simulink library "model_controller"  (R2016b)
settings: Solver=VariableStepAuto  StartTime=0.0  StopTime=10.0  RelTol=1e-3
undefined symbols (not defined in the file or in its folder): acc, ad, dd, jd, jerk, snap, vel
libraries: model_controller x6, motion x1
settings Model: Creator=Dai Luyao  LastModifiedBy=Dai Luyao

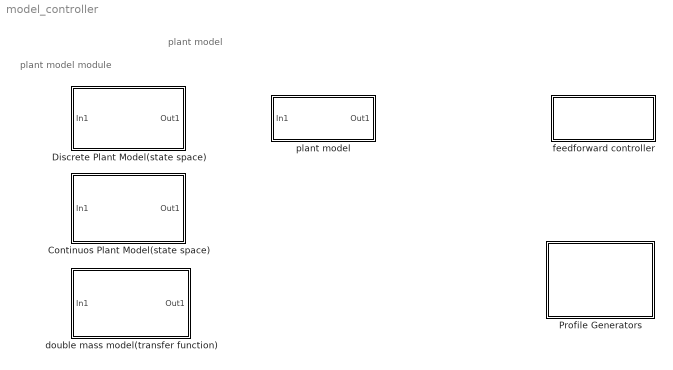
== system model_controller ==
  note: plant model
  note: plant model module
  "Continuos Plant Model(state space) " : Subsystem  mask{A=0, B=0, C=0, D=0}
  Discrete Plant Model(state space) : Subsystem  mask{A_d=0, B_d=0, C_d=0, D_d=0}
      mask prompts: A_d "A"; B_d "B"; C_d "C"; D_d "D"
  Profile Generators : Subsystem
      mask Display: disp('Profile\nGenerators')
  double mass model(transfer function) : Subsystem  mask{m1=0, m2=0, f=0, n=0}
      mask prompts: m1 "mover"; m2 "stage"; f "resonant frequency(Hz)"; n "damping ratio"
  feedforward controller : Subsystem
      mask Display: disp('feedforward controller');
  plant model : Subsystem  BlockChoice=Continuos Plant Model(state space)
      settings: TemplateBlock=self  MemberBlocks=Continuos Plant Model(state space) ,Discrete Plant Model(state space),double mass model(transfer function)

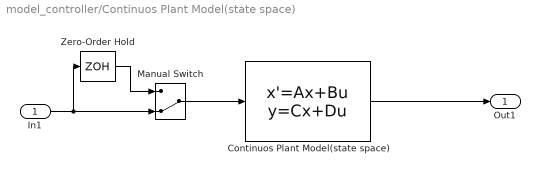
== system model_controller/Continuos Plant Model(state space)  ==
  In1 : Inport
  "Continuos Plant Model(state space) " : StateSpace  A=A  B=B  C=C  D=D  X0=0
  Manual Switch : ManualSwitch  CurrentSetting=0
  Zero-Order Hold : ZeroOrderHold  SampleTime=2e-6
  Out1 : Outport
  wires:
  "Continuos Plant Model(state space) "/1 -> Out1/1
  In1/1 -> Zero-Order Hold/1, Manual Switch/2
  Zero-Order Hold/1 -> Manual Switch/1
  Manual Switch/1 -> "Continuos Plant Model(state space) "/1

== system model_controller/Discrete Plant Model(state space) ==
  In1 : Inport
  Discrete Plant Model(state space) : DiscreteStateSpace  A=A_d  B=B_d  C=B_d  D=D_d  SampleTime=-1
  Out1 : Outport
  wires:
  In1/1 -> Discrete Plant Model(state space)/1
  Discrete Plant Model(state space)/1 -> Out1/1

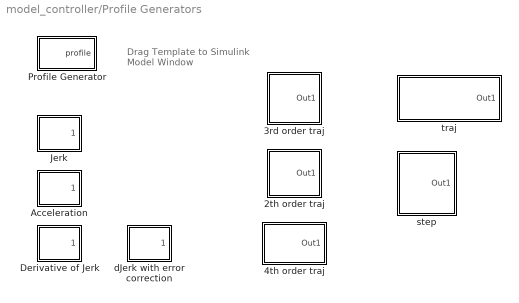
== system model_controller/Profile Generators ==
  note: Drag Template to
      | Simulink Model Window
  2th order traj : Subsystem  mask(2nd Order Profile Generator){t0=0, x=0.06, v=0.25, a=10, Ts=0}
      mask prompts: t0 "Starting time:  t0 [s]"; x "Displacement:  x [m]"; v "Bound on velocity:  vmax [m/s]"; a "Bound on acceleration:  amax [m/s2]"; Ts "Sampling time (0 for continuous):  Ts [s]"
      mask help: 2nd Order Profile Generator
      mask Help: See make2.m and look under mask
  3rd order traj : Subsystem  mask(3d Order Profile Generator){t0=0, x=0.06, v=0.25, a=10, j=800, Ts=0}
      mask prompts: t0 "Starting time:  t0 [s]"; x "Displacement:  x [m]"; v "Bound on velocity:  vmax [m/s]"; a "Bound on acceleration:  amax [m/s2]"; j "Bound on jerk: jmax [m/s3]"; Ts "Sampling time (0 for continuous):  Ts [s]"
      mask help: 3d Order Profile Generator
      mask Help: See make3.m and profile3.m and look under mask
  4th order traj : Subsystem  mask(4th Order Profile Generator){t0=0, x=0.06, v=0.25, a=10, j=800, d=64000, Ts=0}
      mask prompts: t0 "Starting time:  t0 [s]"; x "Displacement:  x [m]"; v "Bound on velocity:  vmax [m/s]"; a "Bound on acceleration:  amax [m/s2]"; j "Bound on jerk: jmax [m/s3]"; d "Bound on derivative of jerk:  dmax [m/s4]"; Ts "Sampling time (0 for continuous):  Ts [s]"
      mask help: 4th Order Profile Generator
      mask Help: See make4.m and profile4.m and look under mask
  Acceleration : Subsystem  mask(2nd Order Profile Generator){t0=.3, x=1, v=1, a=5, Ts=0}
      mask prompts: t0 "Starting time:  t0 [s]"; x "Displacement:  x [m]"; v "Bound on velocity:  vmax [m/s]"; a "Bound on acceleration:  amax [m/s2]"; Ts "Sampling time (0 for continuous):  Ts [s]"
      mask help: 2nd Order Profile Generator
      mask init:
      | [t,ad,aa,tx,a,v,p,tt] = make2(abs(x),v,a,Ts,0);
      | t0=t0-10*eps;
      mask Help: See make2.m and look under mask
      mask Display:
      | plot([0 aa(1,:)+t0],[0 aa(2,:)])
      | text(0.8*(max(aa(1,:))+t0),0,'a\n')
  Derivative of Jerk : Subsystem  mask(4th Order Profile Generator){t0=0.02, x=0.046, v=0.6, a=10, j=800, d=64000, Ts=0}
      mask prompts: t0 "Starting time:  t0 [s]"; x "Displacement:  x [m]"; v "Bound on velocity:  vmax [m/s]"; a "Bound on acceleration:  amax [m/s2]"; j "Bound on jerk: jmax [m/s3]"; d "Bound on derivative of jerk:  dmax [m/s4]"; Ts "Sampling time (0 for continuous):  Ts [s]"
      mask help: 4th Order Profile Generator
      mask init:
      | [t,dd]=make4(abs(x),v,a,j,d,Ts);
      | t0=t0-10*eps;
      | [dj,tx,d,j,a,v,p,tt]=profile4(t,dd(1),0,0);
      mask Help: See make4.m and profile4.m and look under mask
      mask Display:
      | plot([0 dj(1,:)+t0],[0 dj(2,:)])
      | text(0.8*(max(dj(1,:))+t0),0,'d\n')
  Jerk : Subsystem  mask(3d Order Profile Generator){t0=.3, x=1, v=1, a=5, j=50, Ts=0}
      mask prompts: t0 "Starting time:  t0 [s]"; x "Displacement:  x [m]"; v "Bound on velocity:  vmax [m/s]"; a "Bound on acceleration:  amax [m/s2]"; j "Bound on jerk: jmax [m/s3]"; Ts "Sampling time (0 for continuous):  Ts [s]"
      mask help: 3d Order Profile Generator
      mask init:
      | [t,jd]=make3(abs(x),v,a,j,Ts);
      | t0=t0-10*eps;
      | [jj,tx,j,a,v,p,tt]=profile3(t,jd(1),0,0);
      | global constantAccStartTime;
      | global constantAccEndTime;
      | global constantJerkStartTime;
      | global constantJerkEndTime;
      | constantAccStartTime=t0+t(1);
      | constantAccEndTime=constantAccStartTime+t(2);
      | constantJerkStartTime=t0;
      | constantJerkEndTime=t0+0.9*(t(1)-t0);
      mask Help: See make3.m and profile3.m and look under mask
      mask Display:
      | plot([0 jj(1,:)+t0],[0 jj(2,:)])
      | text(0.85*(max(jj(1,:))+t0),0,'j\n')
  Profile Generator : Subsystem  BlockChoice=Acceleration
      settings: TemplateBlock=self  MemberBlocks=Acceleration,Derivative of Jerk,Jerk,dJerk with error correction
  dJerk with error correction : Subsystem  mask(4th Order Profile Generator with quantization error correction){t0=.3, x=1, v=1, a=5, j=50, d=1000, Ts=0, r=10*eps, s=15}
      mask prompts: t0 "Starting time:  t0 [s]"; x "Displacement:  x [m]"; v "Bound on velocity:  vmax [m/s]"; a "Bound on acceleration:  amax [m/s2]"; j "Bound on jerk: jmax [m/s3]"; d "Bound on derivative of jerk:  dmax [m/s4]"; Ts "Sampling time (0 for continuous):  Ts [s]"; r "Resolution of position [m] (default: 10*eps)"; s "Number of decimals for digitized d (default: 15)"
      mask help: 4th Order Profile Generator with quantization error correction
      mask init:
      | if length(r)==0 | length(s)==0
      | 	r=10*eps;
      | 	s=15;
      | end
      | [t,dd]=make4(abs(x),v,a,j,d,Ts,r,s);
      | t0=t0-10*eps;
      | [dj,tx,d,j,a,v,p,tt]=profile4(t,dd(1),0,0);
      mask Help: See make4.m and profile4.m and look under mask
      mask Display:
      | plot([0 dj(1,:)+t0],[0 dj(2,:)])
      | text(0.8*(max(dj(1,:))+t0),0,'d\n')
  step : Subsystem  mask{t=0, v0=0, vf=1, Ts=0}
      mask prompts: t "step time:"; v0 "inital value:"; vf "final value:"; Ts "sample time"
  traj : Subsystem  BlockChoice=2th order traj
      settings: TemplateBlock=self  MemberBlocks=2th order traj,3rd order traj,4th order traj,step

== system model_controller/double mass model(transfer function) ==
  In1 : Inport
  Zero-Order Hold : ZeroOrderHold  SampleTime=-1
  double mass model(transfer function) : Subsystem
  Out1 : Outport
  wires:
  In1/1 -> Zero-Order Hold/1
  double mass model(transfer function)/1(Out1) -> Out1/1
  Zero-Order Hold/1 -> double mass model(transfer function)/1(In1)

== system model_controller/feedforward controller ==
  S-Function : S-Function  FunctionName=adaptiveFeedforward  Parameters=paraNum  SFunctionDeploymentMode=off  EnableBusSupport=off
  acceleration feedforward : Subsystem  mask{snap=snap, jerk=jerk, acc=acc, vel=vel}
      mask prompts: snap "the coefficient of snap feedforward"; jerk "the coefficient of jerk feedforward"; acc "the coefficient of acc feedforward"; vel "the coefficient of vel feedforward"
      mask Display: disp('acceleration feedforward')
  feedforward 4th order : Subsystem  mask{snap=snap, jerk=jerk, acc=acc, vel=vel}
      mask prompts: snap "the coefficient of snap feedforward"; jerk "the coefficient of jerk feedforward"; acc "the coefficient of acc feedforward"; vel "the coefficient of vel feedforward"
      mask Display: disp('acceleration feedforward')
  feedforward controller : Subsystem  BlockChoice=acceleration feedforward
      settings: TemplateBlock=self  MemberBlocks=acceleration feedforward,feedforward 4th order

== system model_controller/plant model ==
  In1 : Inport
  "Continuos Plant Model(state space) " : model_controller/Continuos Plant Model(state space)   A=0  B=0  C=0  D=0
  Out1 : Outport
  wires:
  In1/1 -> "Continuos Plant Model(state space) "/1
  "Continuos Plant Model(state space) "/1 -> Out1/1

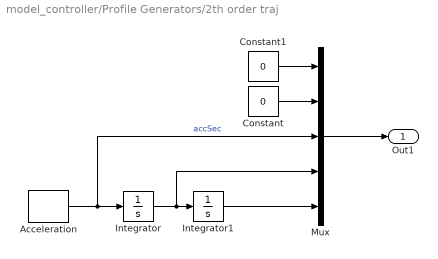
== system model_controller/Profile Generators/2th order traj ==
  Acceleration : model_controller/Profile Generators/Acceleration  t0=t0  x=x  v=v  a=a  Ts=Ts
  Constant : Constant  Value=0
  Constant1 : Constant  Value=0
  Integrator : Integrator
  Integrator1 : Integrator
  Mux : Mux  Inputs=5
  Out1 : Outport
  wires:
  Constant1/1 -> Mux/1
  Constant/1 -> Mux/2
  Integrator1/1 -> Mux/5
  Integrator/1 -> Integrator1/1, Mux/4
  Acceleration/1 -> Integrator/1, Mux/3  "accSec"
  Mux/1 -> Out1/1

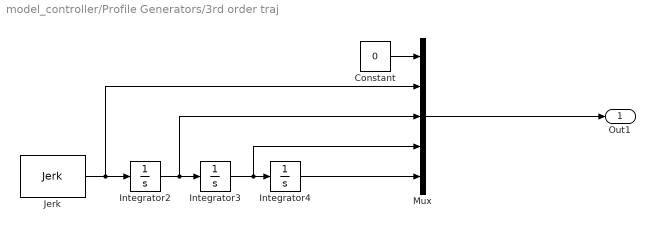
== system model_controller/Profile Generators/3rd order traj ==
  Constant : Constant  Value=0
  Integrator2 : Integrator
  Integrator3 : Integrator
  Integrator4 : Integrator
  Jerk : model_controller/Profile Generators/Jerk  t0=t0  x=x  v=v  a=a  j=j  Ts=Ts
  Mux : Mux  Inputs=5
  Out1 : Outport
  wires:
  Mux/1 -> Out1/1
  Integrator2/1 -> Mux/3, Integrator3/1
  Integrator3/1 -> Mux/4, Integrator4/1
  Jerk/1 -> Mux/2, Integrator2/1
  Integrator4/1 -> Mux/5
  Constant/1 -> Mux/1

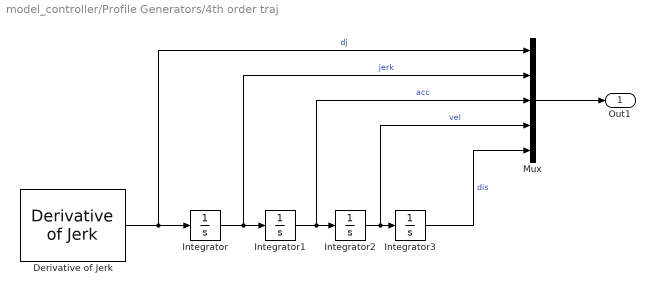
== system model_controller/Profile Generators/4th order traj ==
  Derivative of Jerk : model_controller/Profile Generators/Derivative of Jerk  t0=t0  x=x  v=v  a=a  j=j  d=d  Ts=Ts
  Integrator{,1..3} (4 alike) : Integrator
  Mux : Mux  Inputs=5
  Out1 : Outport
  wires:
  Mux/1 -> Out1/1
  Integrator/1 -> Integrator1/1, Mux/2  "jerk"
  Derivative of Jerk/1 -> Integrator/1, Mux/1  "dj"
  Integrator2/1 -> Integrator3/1, Mux/4  "vel"
  Integrator1/1 -> Integrator2/1, Mux/3  "acc"
  Integrator3/1 -> Mux/5  "dis"

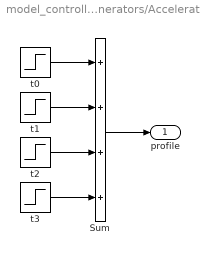
== system model_controller/Profile Generators/Acceleration ==
  Sum : Sum  Inputs=4  SaturateOnIntegerOverflow=on  InputSameDT=on  OutDataTypeStr=Inherit: Same as first input
  t0 : Step  Time=t0  After=ad(1)  SampleTime=0
  t1 : Step  Time=t0+t(1)  After=-ad(1)  SampleTime=0
  t2 : Step  Time=t0+t(1)+t(2)  After=-ad(1)  SampleTime=0
  t3 : Step  Time=t0+2*t(1)+t(2)  After=ad(1)  SampleTime=0
  profile : Outport
  wires:
  t0/1 -> Sum/1
  t1/1 -> Sum/2
  t2/1 -> Sum/3
  t3/1 -> Sum/4
  Sum/1 -> profile/1

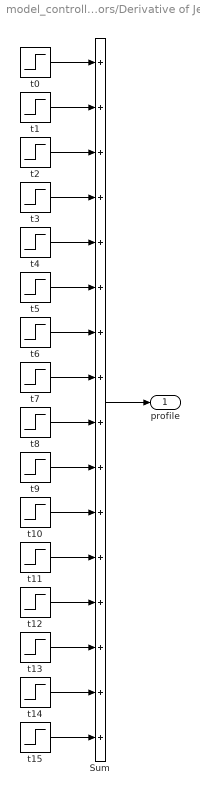
== system model_controller/Profile Generators/Derivative of Jerk ==
  Sum : Sum  Inputs=16  SaturateOnIntegerOverflow=on  InputSameDT=on  OutDataTypeStr=Inherit: Same as first input
  t0 : Step  Time=t0  After=dd(1)  SampleTime=0
  t1 : Step  Time=t0+t(1)  After=-dd(1)  SampleTime=0
  t10 : Step  Time=t0+5*t(1)+3*t(2)+t(3)+t(4)  After=dd(1)  SampleTime=0
  t11 : Step  Time=t0+6*t(1)+3*t(2)+t(3)+t(4)  After=-dd(1)  SampleTime=0
  t12 : Step  Time=t0+6*t(1)+3*t(2)+2*t(3)+t(4)  After=dd(1)  SampleTime=0
  t13 : Step  Time=t0+7*t(1)+3*t(2)+2*t(3)+t(4)  After=-dd(1)  SampleTime=0
  t14 : Step  Time=t0+7*t(1)+4*t(2)+2*t(3)+t(4)  After=-dd(1)  SampleTime=0
  t15 : Step  Time=t0+8*t(1)+4*t(2)+2*t(3)+t(4)  After=dd(1)  SampleTime=0
  t2 : Step  Time=t0+t(1)+t(2)  After=-dd(1)  SampleTime=0
  t3 : Step  Time=t0+2*t(1)+t(2)  After=dd(1)  SampleTime=0
  t4 : Step  Time=t0+2*t(1)+t(2)+t(3)  After=-dd(1)  SampleTime=0
  t5 : Step  Time=t0+3*t(1)+t(2)+t(3)  After=dd(1)  SampleTime=0
  t6 : Step  Time=t0+3*t(1)+2*t(2)+t(3)  After=dd(1)  SampleTime=0
  t7 : Step  Time=t0+4*t(1)+2*t(2)+t(3)  After=-dd(1)  SampleTime=0
  t8 : Step  Time=t0+4*t(1)+2*t(2)+t(3)+t(4)  After=-dd(1)  SampleTime=0
  t9 : Step  Time=t0+5*t(1)+2*t(2)+t(3)+t(4)  After=dd(1)  SampleTime=0
  profile : Outport
  wires:
  t0/1 -> Sum/1
  t1/1 -> Sum/2
  t2/1 -> Sum/3
  t3/1 -> Sum/4
  t4/1 -> Sum/5
  t5/1 -> Sum/6
  t6/1 -> Sum/7
  t7/1 -> Sum/8
  t8/1 -> Sum/9
  t9/1 -> Sum/10
  t10/1 -> Sum/11
  t11/1 -> Sum/12
  t12/1 -> Sum/13
  t13/1 -> Sum/14
  t14/1 -> Sum/15
  t15/1 -> Sum/16
  Sum/1 -> profile/1

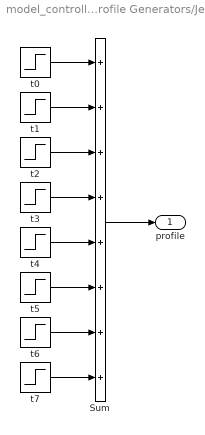
== system model_controller/Profile Generators/Jerk ==
  Sum : Sum  Inputs=8  SaturateOnIntegerOverflow=on  InputSameDT=on  OutDataTypeStr=Inherit: Same as first input
  t0 : Step  Time=t0  After=jd(1)  SampleTime=0
  t1 : Step  Time=t0+t(1)  After=-jd(1)  SampleTime=0
  t2 : Step  Time=t0+t(1)+t(2)  After=-jd(1)  SampleTime=0
  t3 : Step  Time=t0+2*t(1)+t(2)  After=jd(1)  SampleTime=0
  t4 : Step  Time=t0+2*t(1)+t(2)+t(3)  After=-jd(1)  SampleTime=0
  t5 : Step  Time=t0+3*t(1)+t(2)+t(3)  After=jd(1)  SampleTime=0
  t6 : Step  Time=t0+3*t(1)+2*t(2)+t(3)  After=jd(1)  SampleTime=0
  t7 : Step  Time=t0+4*t(1)+2*t(2)+t(3)  After=-jd(1)  SampleTime=0
  profile : Outport
  wires:
  Sum/1 -> profile/1
  t7/1 -> Sum/8
  t6/1 -> Sum/7
  t5/1 -> Sum/6
  t4/1 -> Sum/5
  t3/1 -> Sum/4
  t2/1 -> Sum/3
  t1/1 -> Sum/2
  t0/1 -> Sum/1

== system model_controller/Profile Generators/Profile Generator ==
  Acceleration : motion/Profile Generators/Acceleration  t0=.3  x=1  v=1  a=5  Ts=0
  profile : Outport
  wires:
  Acceleration/1 -> profile/1

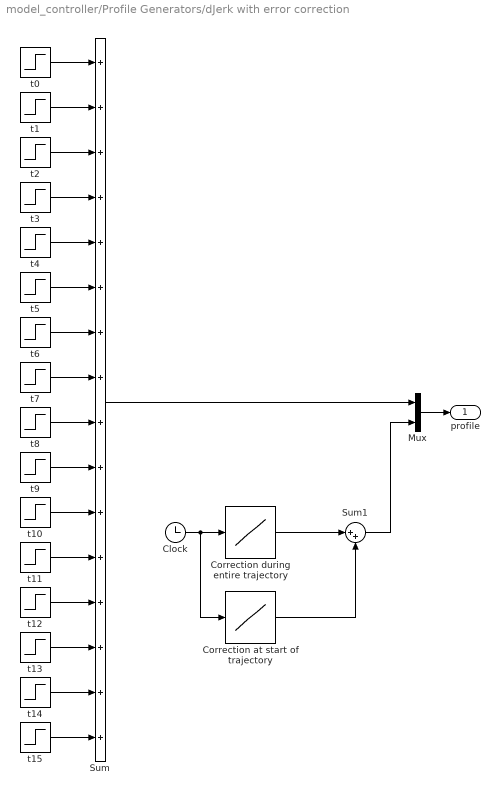
== system model_controller/Profile Generators/dJerk with error correction ==
  Clock : Clock
  Correction at start of trajectory : Lookup  InputValues="[ -1 t0 t0+abs(dd(3))*Ts  2*(t0+8*t(1)+4*t(2)+2*t(3)+t(4)) ]"  Table=[ 0 0 [1 1]*dd(3)*r]  SaturateOnIntegerOverflow=on
  Correction during entire trajectory : Lookup  InputValues="[ -1 t0  t0+8*t(1)+4*t(2)+2*t(3)+t(4)  2*(t0+8*t(1)+4*t(2)+2*t(3)+t(4)) ]"  Table=[0 0 [1 1]*dd(2)*r]  SaturateOnIntegerOverflow=on
  Mux : Mux  Inputs=2
  Sum : Sum  Inputs=16  SaturateOnIntegerOverflow=on  InputSameDT=on  OutDataTypeStr=Inherit: Same as first input
  Sum1 : Sum  Inputs=|++  SaturateOnIntegerOverflow=on  InputSameDT=on  OutDataTypeStr=Inherit: Same as first input
  t0 : Step  Time=t0  After=dd(1)  SampleTime=0
  t1 : Step  Time=t0+t(1)  After=-dd(1)  SampleTime=0
  t10 : Step  Time=t0+5*t(1)+3*t(2)+t(3)+t(4)  After=dd(1)  SampleTime=0
  t11 : Step  Time=t0+6*t(1)+3*t(2)+t(3)+t(4)  After=-dd(1)  SampleTime=0
  t12 : Step  Time=t0+6*t(1)+3*t(2)+2*t(3)+t(4)  After=dd(1)  SampleTime=0
  t13 : Step  Time=t0+7*t(1)+3*t(2)+2*t(3)+t(4)  After=-dd(1)  SampleTime=0
  t14 : Step  Time=t0+7*t(1)+4*t(2)+2*t(3)+t(4)  After=-dd(1)  SampleTime=0
  t15 : Step  Time=t0+8*t(1)+4*t(2)+2*t(3)+t(4)  After=dd(1)  SampleTime=0
  t2 : Step  Time=t0+t(1)+t(2)  After=-dd(1)  SampleTime=0
  t3 : Step  Time=t0+2*t(1)+t(2)  After=dd(1)  SampleTime=0
  t4 : Step  Time=t0+2*t(1)+t(2)+t(3)  After=-dd(1)  SampleTime=0
  t5 : Step  Time=t0+3*t(1)+t(2)+t(3)  After=dd(1)  SampleTime=0
  t6 : Step  Time=t0+3*t(1)+2*t(2)+t(3)  After=dd(1)  SampleTime=0
  t7 : Step  Time=t0+4*t(1)+2*t(2)+t(3)  After=-dd(1)  SampleTime=0
  t8 : Step  Time=t0+4*t(1)+2*t(2)+t(3)+t(4)  After=-dd(1)  SampleTime=0
  t9 : Step  Time=t0+5*t(1)+2*t(2)+t(3)+t(4)  After=dd(1)  SampleTime=0
  profile : Outport
  wires:
  Sum/1 -> Mux/1
  Mux/1 -> profile/1
  t0/1 -> Sum/1
  t1/1 -> Sum/2
  t2/1 -> Sum/3
  t3/1 -> Sum/4
  t4/1 -> Sum/5
  t5/1 -> Sum/6
  t6/1 -> Sum/7
  t7/1 -> Sum/8
  t8/1 -> Sum/9
  t9/1 -> Sum/10
  t10/1 -> Sum/11
  t11/1 -> Sum/12
  t12/1 -> Sum/13
  t13/1 -> Sum/14
  t14/1 -> Sum/15
  t15/1 -> Sum/16
  Clock/1 -> Correction during entire trajectory/1, Correction at start of trajectory/1
  Correction at start of trajectory/1 -> Sum1/2
  Sum1/1 -> Mux/2
  Correction during entire trajectory/1 -> Sum1/1

== system model_controller/Profile Generators/step ==
  Constant : Constant  Value=0
  Mux : Mux  Inputs=5
  Step : Step  Time=t  Before=v0  After=vf  SampleTime=Ts
  Out1 : Outport
  wires:
  Constant/1 -> Mux/1, Mux/4, Mux/3, Mux/2
  Mux/1 -> Out1/1
  Step/1 -> Mux/5

== system model_controller/Profile Generators/traj ==
  2th order traj : model_controller/Profile Generators/2th order traj  t0=0  x=0.06  v=0.25  a=10  Ts=0
  Out1 : Outport
  wires:
  2th order traj/1 -> Out1/1

== system model_controller/double mass model(transfer function)/double mass model(transfer function) ==
  In1 : Inport
  Transfer Fcn : TransferFcn  Denominator=[1 1]
  Out1 : Outport
  wires:
  In1/1 -> Transfer Fcn/1
  Transfer Fcn/1 -> Out1/1

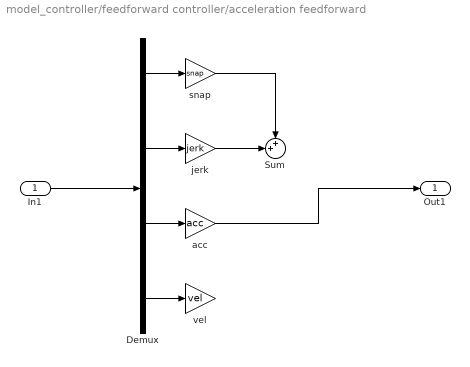
== system model_controller/feedforward controller/acceleration feedforward ==
  In1 : Inport
  Demux : Demux
  Sum : Sum  Inputs=++|
  acc : Gain  Gain=acc
  jerk : Gain  Gain=jerk
  snap : Gain  Gain=snap
  vel : Gain  Gain=vel
  Out1 : Outport
  wires:
  acc/1 -> Out1/1
  snap/1 -> Sum/1
  jerk/1 -> Sum/2
  Demux/4 -> vel/1
  Demux/3 -> acc/1
  Demux/2 -> jerk/1
  Demux/1 -> snap/1
  In1/1 -> Demux/1

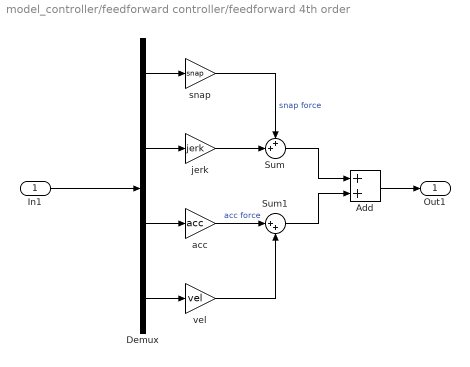
== system model_controller/feedforward controller/feedforward 4th order ==
  In1 : Inport
  Add : Sum
  Demux : Demux
  Sum : Sum  Inputs=++|
  Sum1 : Sum  Inputs=|++
  acc : Gain  Gain=acc
  jerk : Gain  Gain=jerk
  snap : Gain  Gain=snap
  vel : Gain  Gain=vel
  Out1 : Outport
  wires:
  In1/1 -> Demux/1
  Demux/1 -> snap/1
  Demux/2 -> jerk/1
  Demux/3 -> acc/1
  Demux/4 -> vel/1
  jerk/1 -> Sum/2
  snap/1 -> Sum/1  "snap force"
  acc/1 -> Sum1/1  "acc force"
  vel/1 -> Sum1/2
  Sum/1 -> Add/1
  Sum1/1 -> Add/2
  Add/1 -> Out1/1

== system model_controller/feedforward controller/feedforward controller ==
  In1 : Inport
  acceleration feedforward : model_controller/feedforward controller/acceleration feedforward  snap=0  jerk=0  acc=0  vel=0
  Out1 : Outport
  wires:
  In1/1 -> acceleration feedforward/1
  acceleration feedforward/1 -> Out1/1
